simulink model "tren_state_space_model"  (Simulink 8.2)
settings: Solver=ode45  StartTime=0.0  StopTime=1000  RelTol=1e-3
values from neighbouring files (symbols this model uses):
  AAtr = [zeros(17) eye(17) ... (first row only)    [train_state_space_matrices.m]
  BBtr = [zeros(20,8) ... (first row only)    [train_state_space_matrices.m]
  CCtr = zeros(1,34)    [train_state_space_matrices.m]
  DDtr = [zeros(1,8)]    [train_state_space_matrices.m]
  Ltr1y1 = 12.25    [train_katsayi.m]
  Ltr1y2 = 12.25    [train_katsayi.m]
  Ltr2y1 = 1.25    [train_katsayi.m]
  Ltr2y2 = 1.25    [train_katsayi.m]
  Ltr3y1 = 1.25    [train_katsayi.m]
  Ltr3y2 = 1.25    [train_katsayi.m]
  Vtr = 40    [train_katsayi.m]
undefined symbols (not defined in the file or in its folder): get
libraries: dspxfrm3 x1, dspsnks4 x1, dspsigops x1
settings Model: Creator=DOAN  LastModifiedBy=oguzhan
settings DataIOCC: SignalLoggingSaveFormat=Dataset
settings OptimizationCC: ExpressionDepthLimit=128
settings DebuggingCC: FcnCallInpInsideContextMsg=EnableAllAsError  StateNameClashWarn=none
settings GRTTargetCC: CombineOutputUpdateFcns=on  GRTInterface=off

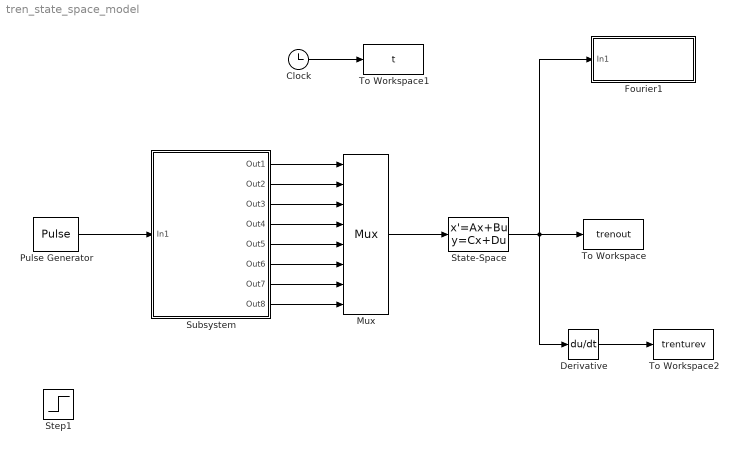
== system tren_state_space_model ==
  Clock : Clock
  Derivative : Derivative
  Fourier1 : Subsystem
  Mux : Mux  Inputs=8
  Pulse Generator : DiscretePulseGenerator  PulseType=Time based  Amplitude=-0.01  Period=0.5  PulseWidth=0.025
  State-Space : StateSpace  A=AAtr  B=BBtr  C=CCtr  D=DDtr  X0=0
  Step1 : Step  SampleTime=0
  Subsystem : Subsystem
  To Workspace : ToWorkspace  VariableName=trenout  SampleTime=-1
  To Workspace1 : ToWorkspace  VariableName=t  SampleTime=-1
  To Workspace2 : ToWorkspace  VariableName=trenturev  SampleTime=-1
  wires:
  Subsystem/1(Out1) -> Mux/1
  Subsystem/2(Out2) -> Mux/2
  Subsystem/3(Out3) -> Mux/3
  Subsystem/4(Out4) -> Mux/4
  Subsystem/5(Out5) -> Mux/5
  Subsystem/6(Out6) -> Mux/6
  Subsystem/7(Out7) -> Mux/7
  Subsystem/8(Out8) -> Mux/8
  Mux/1 -> State-Space/1
  State-Space/1 -> Fourier1/1(In1), Derivative/1, To Workspace/1
  Clock/1 -> To Workspace1/1
  Pulse Generator/1 -> Subsystem/1(In1)
  Derivative/1 -> To Workspace2/1

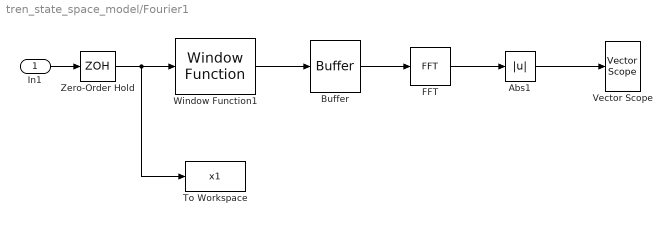
== system tren_state_space_model/Fourier1 ==
  In1 : Inport
  Abs1 : Abs
  Buffer : Buffer  N=2^10  TreatMby1Signals=One channel
  FFT : dspxfrm3/FFT  CompMethod=Table lookup  TableOpt=NEW  TableOptActive=Speed  BitRevOrder=off  InheritFFTLength=on  FFTLength=2048  RowConvenienceOn=on  FFTImplementation=FFTW  SkipNorm=on  firstCoeffDataTypeStr=Inherit: Same word length as input  firstCoeffLastDataTypeStr=Inherit: Same word length as input  outputMin=[]  outputMax=[]  roundingMode=Floor  overflowMode=off
  To Workspace : ToWorkspace  VariableName=x1  SampleTime=-1
  Vector Scope : dspsnks4/Vector Scope  ScopeProperties=on  Domain=Frequency  HorizSpan=1  DisplayProperties=off  AxisGrid=on  Memory=off  FrameNumber=on  AxisLegend=off  AxisZoom=off  OpenScopeAtSimStart=on  OpenScopeImmediately=off  FigPos=get(0,'defaultfigureposition')  AxisProperties=off  XUnits=rad/sec  XRange=[0...Fs/2]  InheritXIncr=on  XIncr=1  XLabel=Time  XLimit=Auto  XMin=0  XMax=300  XStart=0  YUnits=dB  YLabel=Amplitude  LineProperties=off  XAxisParamsVer=6.9
      settings: YMin=-100  YMax=-50
  Window Function1 : dspsigops/Window Function  winmode=Apply window to input  wintype=Hamming  sampmode=Continuous  samptime=1  N=64  Rs=50  beta=10  winsamp=Symmetric  UserWindow=hamming  OptParams=off  UserParams={'symmetric'}  RowConvenienceOn=on  dataType=double  isSigned=on  wordLen=16  udDataType=sfix(16)  fracBitsMode=Best precision  numFracBits=15  roundingMode=Floor  overflowMode=off  numSidelobes=4  sidelobeLevel=-30
  Zero-Order Hold : ZeroOrderHold  SampleTime=1/100
  wires:
  Abs1/1 -> Vector Scope/1
  Window Function1/1 -> Buffer/1
  Zero-Order Hold/1 -> Window Function1/1, To Workspace/1
  In1/1 -> Zero-Order Hold/1
  FFT/1 -> Abs1/1
  Buffer/1 -> FFT/1

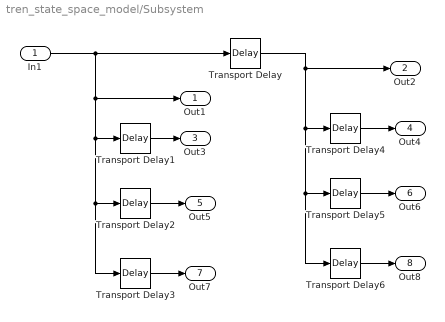
== system tren_state_space_model/Subsystem ==
  In1 : Inport
  Transport Delay : TransportDelay  DelayTime=0.001
  Transport Delay1 : TransportDelay  DelayTime=(Ltr2y1+Ltr2y2)/Vtr
  Transport Delay2 : TransportDelay  DelayTime=(Ltr2y1+Ltr1y1+Ltr1y2-Ltr3y1)/Vtr
  Transport Delay3 : TransportDelay  DelayTime=(Ltr2y1+Ltr1y1+Ltr1y2+Ltr3y2)/Vtr
  Transport Delay4 : TransportDelay  DelayTime=(Ltr2y1+Ltr2y2)/Vtr
  Transport Delay5 : TransportDelay  DelayTime=(Ltr2y1+Ltr1y1+Ltr1y2-Ltr3y1)/Vtr
  Transport Delay6 : TransportDelay  DelayTime=(Ltr2y1+Ltr1y1+Ltr1y2+Ltr3y2)/Vtr
  Out1 : Outport
  Out2 : Outport  Port=2
  Out3 : Outport  Port=3
  Out4 : Outport  Port=4
  Out5 : Outport  Port=5
  Out6 : Outport  Port=6
  Out7 : Outport  Port=7
  Out8 : Outport  Port=8
  wires:
  In1/1 -> Transport Delay/1, Out1/1, Transport Delay1/1, Transport Delay2/1, Transport Delay3/1
  Transport Delay/1 -> Out2/1, Transport Delay6/1, Transport Delay5/1, Transport Delay4/1
  Transport Delay1/1 -> Out3/1
  Transport Delay2/1 -> Out5/1
  Transport Delay3/1 -> Out7/1
  Transport Delay4/1 -> Out4/1
  Transport Delay5/1 -> Out6/1
  Transport Delay6/1 -> Out8/1
